simulink model "CL_controller_euler_v1"  (R2016b)
settings: Solver=ode45  StartTime=0.0  StopTime=10.0  FixedStep=1/512  RelTol=1e-3
undefined symbols (not defined in the file): pars
settings Model: Creator=kkajak  LastModifiedBy=Karl

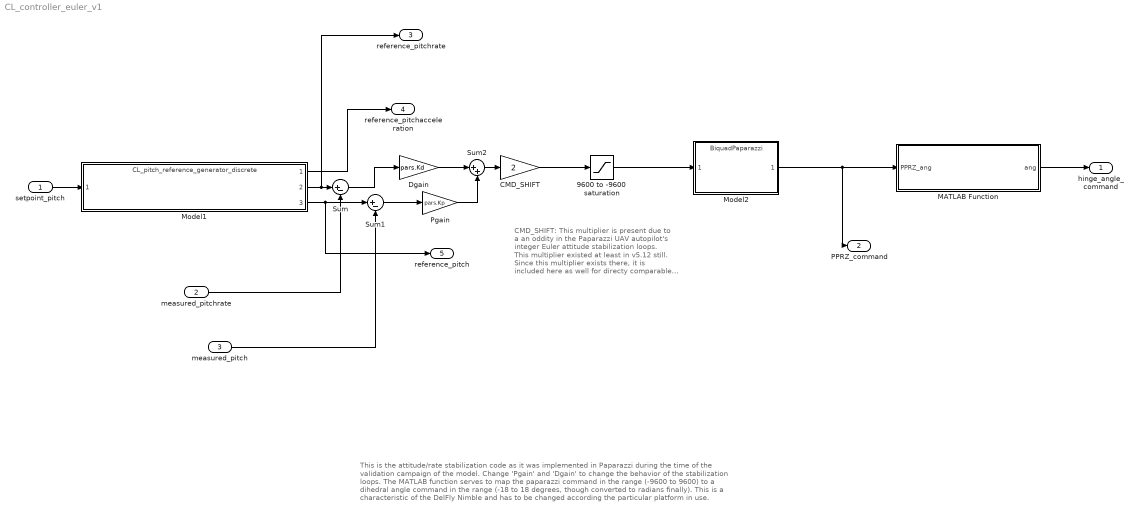
== system CL_controller_euler_v1 ==
  note: This is the attitude/rate stabilization code as it was implemented in Paparazzi during the time of the validation campaign of the model.
      | Change 'Pgain' and 'Dgain' to change the behavior of the stabilization loops. The MATLAB function serves to map the paparazzi command
      | in the range (-9600 to 9600) to a dihedral angle command in the range (-18 to 18 degrees, though converted to radians finally). This is a
      | characteristic of the DelFly Nimble and has to be changed according the particular platform in use.
  note: CMD_SHIFT:
      | This multiplier is present due to a an oddity in the Paparazzi UAV
      | autopilot's integer Euler attitude stabilization loops. This multiplier existed
      | at least in v5.12 still. Since this multiplier exists there, it is included here as
      | well for directy comparable gains. It was handy for our work, but it need not
      | exist for the general user of the model.
  setpoint_pitch : Inport  SampleTime=1/512
  measured_pitchrate : Inport  Port=2
  measured_pitch : Inport  Port=3
  9600 to -9600 saturation : Saturate  UpperLimit=9600  LowerLimit=-9600
  CMD_SHIFT : Gain  Gain=2
  Dgain : Gain  Gain=pars.Kd
  MATLAB Function : MATLAB Function  TreatAsAtomicUnit=on
  Model1 : ModelReference  ModelNameDialog=CL_pitch_reference_generator_discrete.slx  SimulationMode=Normal  ModelReferenceVersion=1.11
  Model2 : ModelReference  ModelNameDialog=BiquadPaparazzi  SimulationMode=Normal  ModelReferenceVersion=1.4
  Pgain : Gain  Gain=pars.Kp
  Sum : Sum  Inputs=|+-
  Sum1 : Sum  Inputs=|+-
  Sum2 : Sum  Inputs=|++
  hinge_angle_command : Outport  SampleTime=1/512
  PPRZ_command : Outport  Port=2
  reference_pitchrate : Outport  Port=3
  reference_pitchacceleration : Outport  Port=4
  reference_pitch : Outport  Port=5
  wires:
  Sum2/1 -> CMD_SHIFT/1
  Model1/2 -> reference_pitchrate/1, Sum/1
  Sum/1 -> Dgain/1
  Sum1/1 -> Pgain/1
  Dgain/1 -> Sum2/1
  Pgain/1 -> Sum2/2
  Model1/3 -> reference_pitch/1, Sum1/1
  setpoint_pitch/1 -> Model1/1
  measured_pitchrate/1 -> Sum/2
  measured_pitch/1 -> Sum1/2
  MATLAB Function/1(ang) -> hinge_angle_command/1
  Model1/1 -> reference_pitchacceleration/1
  Model2/1 -> PPRZ_command/1, MATLAB Function/1(PPRZ_ang)
  CMD_SHIFT/1 -> 9600 to -9600 saturation/1
  9600 to -9600 saturation/1 -> Model2/1

== matlab function CL_controller_euler_v1/MATLAB Function ==
  data: PPRZ_ang input; ang output
function ang  = fcn(PPRZ_ang)
ang = ((PPRZ_ang)/9600*18)/180*pi;
